simulink model "r2_c8n856m1k_wo_pfb"  (R2013a)
(part 2 of 31)

      | elseif strcmp(mode, 'fields of arbitrary size')
      |     current_names = textscan(strtrim(strrep(strrep(get_param(blk, 'names'), ']', ''), '[', '')), '%s');
      |     current_names = current_names{1};
      |     numios = length(current_names);
      |     if length(current_types) ~= numios,
      |         error('%d field names specified, but %d types?', numios, length(current_types));
      |     end
      | end
      | problem = 0;
      | for ctr = 1 : numios,
      |     t = current_types(ctr);
      |     if (t < 0) || (t > 2),
      |         problem = t;
      |         ctr = numios + 1;
      |     end
      | end
      | if problem ~= 0,
      |     error('Type cannot be %i, must be 0, 1 or 2.', problem);
      | end
      mask Callback bin_pts:
      | blk = gcb;
      | mode = get_param(blk, 'mode');
      | current_bins = eval(get_param(blk, 'bin_pts'));
      | if (strcmp(mode, 'one value') || strcmp(mode, 'fields of equal size')) && (length(current_bins) > 1),
      |     error('Only one binary pt may be specified for this mode.');
      | elseif strcmp(mode, 'fields of arbitrary size')
      |     current_names = textscan(strtrim(strrep(strrep(get_param(blk, 'names'), ']', ''), '[', '')), '%s');
      |     current_names = current_names{1};
      |     numios = length(current_names);
      |     if length(current_bins) ~= numios,
      |         error('%d field names specified, but %d binary pts?', numios, length(current_bins));
      |     end
      | end
  sync_timestamp_msw : Subsystem  Tag=xps:sw_reg  AncestorBlock=xps_library/software register  mask(swreg){mode=one value, io_dir=To Processor, io_delay=0, sample_period=1, names=reg, bitwidths=32, arith_types=0, bin_pts=0, sim_port=off, show_format=on}
      mask prompts: io_dir "I/O direction"; io_delay "I/O delay"; sample_period "Sample period"; names "Name:"; bitwidths "Bitwidth:"; arith_types "Type (ufix=0, fix=1, bool=2):"; bin_pts "Binary pt:"; sim_port "Provide sim input/output?"; show_format "Print format string?"
      mask init:
      | swreg_init(gcb)
      settings: AttributesFormatString=1output:uf32.0,
      mask TypeOptions mode: one value | fields of equal size | fields of arbitrary size
      mask Callback mode: swreg_cb(gcb);
      mask TypeOptions io_dir: To Processor | From Processor
      mask Callback io_dir:
      | mask_enables = get_param(gcb, 'MaskEnables');
      | mask_names = get_param(gcb, 'MaskNames');
      | if strcmp(get_param(gcb, 'io_dir'), 'To Processor'),
      |     mask_enables{ismember(mask_names, 'sample_period')} = 'off';
      | else
      |     mask_enables{ismember(mask_names, 'sample_period')} = 'on';
      | end
      | set_param(gcb, 'MaskEnables', mask_enables);
      mask Callback bitwidths:
      | blk = gcb;
      | mode = get_param(blk, 'mode');
      | current_widths = eval(get_param(blk, 'bitwidths'));
      | if (strcmp(mode, 'one value') || strcmp(mode, 'fields of equal size')) && (length(current_widths) > 1),
      |     error('Only one width may be specified for this mode.');
      | elseif strcmp(mode, 'fields of arbitrary size')
      |     current_names = textscan(strtrim(strrep(strrep(get_param(blk, 'names'), ']', ''), '[', '')), '%s');
      |     current_names = current_names{1};
      |     numios = length(current_names);
      |     if length(current_widths) ~= numios,
      |         error('%d field names specified, but %d widths?', numios, length(current_widths));
      |     end
      | end
      | total_width = 0;
      | for ctr = 1 : length(current_widths),
      |     total_width = total_width + current_widths(ctr);
      | end
      | if total_width > 32,
      |     error('Total width must be 32 or less, set to %d.', total_width);
      | end
      mask Callback arith_types:
      | blk = gcb;
      | mode = get_param(blk, 'mode');
      | current_types = eval(get_param(blk, 'arith_types'));
      | numios = length(current_types);
      | if (strcmp(mode, 'one value') || strcmp(mode, 'fields of equal size')) && (length(current_types) > 1),
      |     error('Only one type may be specified for this mode.');
      | elseif strcmp(mode, 'fields of arbitrary size')
      |     current_names = textscan(strtrim(strrep(strrep(get_param(blk, 'names'), ']', ''), '[', '')), '%s');
      |     current_names = current_names{1};
      |     numios = length(current_names);
      |     if length(current_types) ~= numios,
      |         error('%d field names specified, but %d types?', numios, length(current_types));
      |     end
      | end
      | problem = 0;
      | for ctr = 1 : numios,
      |     t = current_types(ctr);
      |     if (t < 0) || (t > 2),
      |         problem = t;
      |         ctr = numios + 1;
      |     end
      | end
      | if problem ~= 0,
      |     error('Type cannot be %i, must be 0, 1 or 2.', problem);
      | end
      mask Callback bin_pts:
      | blk = gcb;
      | mode = get_param(blk, 'mode');
      | current_bins = eval(get_param(blk, 'bin_pts'));
      | if (strcmp(mode, 'one value') || strcmp(mode, 'fields of equal size')) && (length(current_bins) > 1),
      |     error('Only one binary pt may be specified for this mode.');
      | elseif strcmp(mode, 'fields of arbitrary size')
      |     current_names = textscan(strtrim(strrep(strrep(get_param(blk, 'names'), ']', ''), '[', '')), '%s');
      |     current_names = current_names{1};
      |     numios = length(current_names);
      |     if length(current_bins) ~= numios,
      |         error('%d field names specified, but %d binary pts?', numios, length(current_bins));
      |     end
      | end
  timestep_ages : Subsystem  Tag=xps:sw_reg  AncestorBlock=xps_library/software register  mask(swreg){mode=fields of equal size, io_dir=To Processor, io_delay=0, sample_period=1, names=[future past], bitwidths=16, arith_types=0, bin_pts=0, sim_port=off, show_format=on}
      mask prompts: io_dir "I/O direction"; io_delay "I/O delay"; sample_period "Sample period"; names "Names [msb ... lsb]:"; bitwidths "Bitwidth:"; arith_types "Type (ufix=0, fix=1, bool=2):"; bin_pts "Binary pt:"; sim_port "Provide sim input/output?"; show_format "Print format string?"
      mask init:
      | swreg_init(gcb)
      settings: AttributesFormatString=2 outputs:uf16.0,uf16.0,
      mask TypeOptions mode: one value | fields of equal size | fields of arbitrary size
      mask Callback mode: swreg_cb(gcb);
      mask TypeOptions io_dir: To Processor | From Processor
      mask Callback io_dir:
      | mask_enables = get_param(gcb, 'MaskEnables');
      | mask_names = get_param(gcb, 'MaskNames');
      | if strcmp(get_param(gcb, 'io_dir'), 'To Processor'),
      |     mask_enables{ismember(mask_names, 'sample_period')} = 'off';
      | else
      |     mask_enables{ismember(mask_names, 'sample_period')} = 'on';
      | end
      | set_param(gcb, 'MaskEnables', mask_enables);
      mask Callback bitwidths:
      | blk = gcb;
      | mode = get_param(blk, 'mode');
      | current_widths = eval(get_param(blk, 'bitwidths'));
      | if (strcmp(mode, 'one value') || strcmp(mode, 'fields of equal size')) && (length(current_widths) > 1),
      |     error('Only one width may be specified for this mode.');
      | elseif strcmp(mode, 'fields of arbitrary size')
      |     current_names = textscan(strtrim(strrep(strrep(get_param(blk, 'names'), ']', ''), '[', '')), '%s');
      |     current_names = current_names{1};
      |     numios = length(current_names);
      |     if length(current_widths) ~= numios,
      |         error('%d field names specified, but %d widths?', numios, length(current_widths));
      |     end
      | end
      | total_width = 0;
      | for ctr = 1 : length(current_widths),
      |     total_width = total_width + current_widths(ctr);
      | end
      | if total_width > 32,
      |     error('Total width must be 32 or less, set to %d.', total_width);
      | end
      mask Callback arith_types:
      | blk = gcb;
      | mode = get_param(blk, 'mode');
      | current_types = eval(get_param(blk, 'arith_types'));
      | numios = length(current_types);
      | if (strcmp(mode, 'one value') || strcmp(mode, 'fields of equal size')) && (length(current_types) > 1),
      |     error('Only one type may be specified for this mode.');
      | elseif strcmp(mode, 'fields of arbitrary size')
      |     current_names = textscan(strtrim(strrep(strrep(get_param(blk, 'names'), ']', ''), '[', '')), '%s');
      |     current_names = current_names{1};
      |     numios = length(current_names);
      |     if length(current_types) ~= numios,
      |         error('%d field names specified, but %d types?', numios, length(current_types));
      |     end
      | end
      | problem = 0;
      | for ctr = 1 : numios,
      |     t = current_types(ctr);
      |     if (t < 0) || (t > 2),
      |         problem = t;
      |         ctr = numios + 1;
      |     end
      | end
      | if problem ~= 0,
      |     error('Type cannot be %i, must be 0, 1 or 2.', problem);
      | end
      mask Callback bin_pts:
      | blk = gcb;
      | mode = get_param(blk, 'mode');
      | current_bins = eval(get_param(blk, 'bin_pts'));
      | if (strcmp(mode, 'one value') || strcmp(mode, 'fields of equal size')) && (length(current_bins) > 1),
      |     error('Only one binary pt may be specified for this mode.');
      | elseif strcmp(mode, 'fields of arbitrary size')
      |     current_names = textscan(strtrim(strrep(strrep(get_param(blk, 'names'), ']', ''), '[', '')), '%s');
      |     current_names = current_names{1};
      |     numios = length(current_names);
      |     if length(current_bins) ~= numios,
      |         error('%d field names specified, but %d binary pts?', numios, length(current_bins));
      |     end
      | end
  tl_unpack_flags : Subsystem  mask(timed_latch){n_bits_time=48, n_bits_offset=(9+3), n_bits_counters=8}
      mask prompts: n_bits_time "Total time resolution (bits)"; n_bits_offset "Offset from lsb for comparison"; n_bits_counters "Bits in status counters"
      mask help:
      | Latches load_value when armed and current_time matches requested time.
      | current_time should be in ADC samples.
      mask init:
      | set_param([gcb,'/status'], 'bitwidths', mat2str([1, repmat(n_bits_counters, 1, 2)]));
      mask Help:
      | When armed, will latch new value when current time matches the time
      | specified. The input time should be in samples and mask settings allow
      | a portion of this to be compared to cater for quantization. Arm and latch
      | counts allow the current state, pending and missed latch events to be
      | determined.
  tmiss_ctr : Subsystem  Tag=xps:sw_reg  AncestorBlock=xps_library/software register  mask(swreg){mode=fields of equal size, io_dir=To Processor, io_delay=0, sample_period=1, names=[p0 p1], bitwidths=16, arith_types=0, bin_pts=0, sim_port=off, show_format=on}
      mask prompts: io_dir "I/O direction"; io_delay "I/O delay"; sample_period "Sample period"; names "Names [msb ... lsb]:"; bitwidths "Bitwidth:"; arith_types "Type (ufix=0, fix=1, bool=2):"; bin_pts "Binary pt:"; sim_port "Provide sim input/output?"; show_format "Print format string?"
      mask init:
      | swreg_init(gcb)
      settings: AttributesFormatString=2 outputs:uf16.0,uf16.0,
      mask TypeOptions mode: one value | fields of equal size | fields of arbitrary size
      mask Callback mode: swreg_cb(gcb);
      mask TypeOptions io_dir: To Processor | From Processor
      mask Callback io_dir:
      | mask_enables = get_param(gcb, 'MaskEnables');
      | mask_names = get_param(gcb, 'MaskNames');
      | if strcmp(get_param(gcb, 'io_dir'), 'To Processor'),
      |     mask_enables{ismember(mask_names, 'sample_period')} = 'off';
      | else
      |     mask_enables{ismember(mask_names, 'sample_period')} = 'on';
      | end
      | set_param(gcb, 'MaskEnables', mask_enables);
      mask Callback bitwidths:
      | blk = gcb;
      | mode = get_param(blk, 'mode');
      | current_widths = eval(get_param(blk, 'bitwidths'));
      | if (strcmp(mode, 'one value') || strcmp(mode, 'fields of equal size')) && (length(current_widths) > 1),
      |     error('Only one width may be specified for this mode.');
      | elseif strcmp(mode, 'fields of arbitrary size')
      |     current_names = textscan(strtrim(strrep(strrep(get_param(blk, 'names'), ']', ''), '[', '')), '%s');
      |     current_names = current_names{1};
      |     numios = length(current_names);
      |     if length(current_widths) ~= numios,
      |         error('%d field names specified, but %d widths?', numios, length(current_widths));
      |     end
      | end
      | total_width = 0;
      | for ctr = 1 : length(current_widths),
      |     total_width = total_width + current_widths(ctr);
      | end
      | if total_width > 32,
      |     error('Total width must be 32 or less, set to %d.', total_width);
      | end
      mask Callback arith_types:
      | blk = gcb;
      | mode = get_param(blk, 'mode');
      | current_types = eval(get_param(blk, 'arith_types'));
      | numios = length(current_types);
      | if (strcmp(mode, 'one value') || strcmp(mode, 'fields of equal size')) && (length(current_types) > 1),
      |     error('Only one type may be specified for this mode.');
      | elseif strcmp(mode, 'fields of arbitrary size')
      |     current_names = textscan(strtrim(strrep(strrep(get_param(blk, 'names'), ']', ''), '[', '')), '%s');
      |     current_names = current_names{1};
      |     numios = length(current_names);
      |     if length(current_types) ~= numios,
      |         error('%d field names specified, but %d types?', numios, length(current_types));
      |     end
      | end
      | problem = 0;
      | for ctr = 1 : numios,
      |     t = current_types(ctr);
      |     if (t < 0) || (t > 2),
      |         problem = t;
      |         ctr = numios + 1;
      |     end
      | end
      | if problem ~= 0,
      |     error('Type cannot be %i, must be 0, 1 or 2.', problem);
      | end
      mask Callback bin_pts:
      | blk = gcb;
      | mode = get_param(blk, 'mode');
      | current_bins = eval(get_param(blk, 'bin_pts'));
      | if (strcmp(mode, 'one value') || strcmp(mode, 'fields of equal size')) && (length(current_bins) > 1),
      |     error('Only one binary pt may be specified for this mode.');
      | elseif strcmp(mode, 'fields of arbitrary size')
      |     current_names = textscan(strtrim(strrep(strrep(get_param(blk, 'names'), ']', ''), '[', '')), '%s');
      |     current_names = current_names{1};
      |     numios = length(current_names);
      |     if length(current_bins) ~= numios,
      |         error('%d field names specified, but %d binary pts?', numios, length(current_bins));
      |     end
      | end
  tmiss_p0 : Subsystem  Tag=xps:sw_reg  AncestorBlock=xps_library/software register  mask(swreg){mode=one value, io_dir=To Processor, io_delay=0, sample_period=1, names=reg, bitwidths=32, arith_types=0, bin_pts=0, sim_port=off, show_format=on}
      mask prompts: io_dir "I/O direction"; io_delay "I/O delay"; sample_period "Sample period"; names "Name:"; bitwidths "Bitwidth:"; arith_types "Type (ufix=0, fix=1, bool=2):"; bin_pts "Binary pt:"; sim_port "Provide sim input/output?"; show_format "Print format string?"
      mask init:
      | swreg_init(gcb)
      settings: AttributesFormatString=1output:uf32.0,
      mask TypeOptions mode: one value | fields of equal size | fields of arbitrary size
      mask Callback mode: swreg_cb(gcb);
      mask TypeOptions io_dir: To Processor | From Processor
      mask Callback io_dir:
      | mask_enables = get_param(gcb, 'MaskEnables');
      | mask_names = get_param(gcb, 'MaskNames');
      | if strcmp(get_param(gcb, 'io_dir'), 'To Processor'),
      |     mask_enables{ismember(mask_names, 'sample_period')} = 'off';
      | else
      |     mask_enables{ismember(mask_names, 'sample_period')} = 'on';
      | end
      | set_param(gcb, 'MaskEnables', mask_enables);
      mask Callback bitwidths:
      | blk = gcb;
      | mode = get_param(blk, 'mode');
      | current_widths = eval(get_param(blk, 'bitwidths'));
      | if (strcmp(mode, 'one value') || strcmp(mode, 'fields of equal size')) && (length(current_widths) > 1),
      |     error('Only one width may be specified for this mode.');
      | elseif strcmp(mode, 'fields of arbitrary size')
      |     current_names = textscan(strtrim(strrep(strrep(get_param(blk, 'names'), ']', ''), '[', '')), '%s');
      |     current_names = current_names{1};
      |     numios = length(current_names);
      |     if length(current_widths) ~= numios,
      |         error('%d field names specified, but %d widths?', numios, length(current_widths));
      |     end
      | end
      | total_width = 0;
      | for ctr = 1 : length(current_widths),
      |     total_width = total_width + current_widths(ctr);
      | end
      | if total_width > 32,
      |     error('Total width must be 32 or less, set to %d.', total_width);
      | end
      mask Callback arith_types:
      | blk = gcb;
      | mode = get_param(blk, 'mode');
      | current_types = eval(get_param(blk, 'arith_types'));
      | numios = length(current_types);
      | if (strcmp(mode, 'one value') || strcmp(mode, 'fields of equal size')) && (length(current_types) > 1),
      |     error('Only one type may be specified for this mode.');
      | elseif strcmp(mode, 'fields of arbitrary size')
      |     current_names = textscan(strtrim(strrep(strrep(get_param(blk, 'names'), ']', ''), '[', '')), '%s');
      |     current_names = current_names{1};
      |     numios = length(current_names);
      |     if length(current_types) ~= numios,
      |         error('%d field names specified, but %d types?', numios, length(current_types));
      |     end
      | end
      | problem = 0;
      | for ctr = 1 : numios,
      |     t = current_types(ctr);
      |     if (t < 0) || (t > 2),
      |         problem = t;
      |         ctr = numios + 1;
      |     end
      | end
      | if problem ~= 0,
      |     error('Type cannot be %i, must be 0, 1 or 2.', problem);
      | end
      mask Callback bin_pts:
      | blk = gcb;
      | mode = get_param(blk, 'mode');
      | current_bins = eval(get_param(blk, 'bin_pts'));
      | if (strcmp(mode, 'one value') || strcmp(mode, 'fields of equal size')) && (length(current_bins) > 1),
      |     error('Only one binary pt may be specified for this mode.');
      | elseif strcmp(mode, 'fields of arbitrary size')
      |     current_names = textscan(strtrim(strrep(strrep(get_param(blk, 'names'), ']', ''), '[', '')), '%s');
      |     current_names = current_names{1};
      |     numios = length(current_names);
      |     if length(current_bins) ~= numios,
      |         error('%d field names specified, but %d binary pts?', numios, length(current_bins));
      |     end
      | end
  tmiss_p1 : Subsystem  Tag=xps:sw_reg  AncestorBlock=xps_library/software register  mask(swreg){mode=one value, io_dir=To Processor, io_delay=0, sample_period=1, names=reg, bitwidths=32, arith_types=0, bin_pts=0, sim_port=off, show_format=on}
      mask prompts: io_dir "I/O direction"; io_delay "I/O delay"; sample_period "Sample period"; names "Name:"; bitwidths "Bitwidth:"; arith_types "Type (ufix=0, fix=1, bool=2):"; bin_pts "Binary pt:"; sim_port "Provide sim input/output?"; show_format "Print format string?"
      mask init:
      | swreg_init(gcb)
      settings: AttributesFormatString=1output:uf32.0,
      mask TypeOptions mode: one value | fields of equal size | fields of arbitrary size
      mask Callback mode: swreg_cb(gcb);
      mask TypeOptions io_dir: To Processor | From Processor
      mask Callback io_dir:
      | mask_enables = get_param(gcb, 'MaskEnables');
      | mask_names = get_param(gcb, 'MaskNames');
      | if strcmp(get_param(gcb, 'io_dir'), 'To Processor'),
      |     mask_enables{ismember(mask_names, 'sample_period')} = 'off';
      | else
      |     mask_enables{ismember(mask_names, 'sample_period')} = 'on';
      | end
      | set_param(gcb, 'MaskEnables', mask_enables);
      mask Callback bitwidths:
      | blk = gcb;
      | mode = get_param(blk, 'mode');
      | current_widths = eval(get_param(blk, 'bitwidths'));
      | if (strcmp(mode, 'one value') || strcmp(mode, 'fields of equal size')) && (length(current_widths) > 1),
      |     error('Only one width may be specified for this mode.');
      | elseif strcmp(mode, 'fields of arbitrary size')
      |     current_names = textscan(strtrim(strrep(strrep(get_param(blk, 'names'), ']', ''), '[', '')), '%s');
      |     current_names = current_names{1};
      |     numios = length(current_names);
      |     if length(current_widths) ~= numios,
      |         error('%d field names specified, but %d widths?', numios, length(current_widths));
      |     end
      | end
      | total_width = 0;
      | for ctr = 1 : length(current_widths),
      |     total_width = total_width + current_widths(ctr);
      | end
      | if total_width > 32,
      |     error('Total width must be 32 or less, set to %d.', total_width);
      | end
      mask Callback arith_types:
      | blk = gcb;
      | mode = get_param(blk, 'mode');
      | current_types = eval(get_param(blk, 'arith_types'));
      | numios = length(current_types);
      | if (strcmp(mode, 'one value') || strcmp(mode, 'fields of equal size')) && (length(current_types) > 1),
      |     error('Only one type may be specified for this mode.');
      | elseif strcmp(mode, 'fields of arbitrary size')
      |     current_names = textscan(strtrim(strrep(strrep(get_param(blk, 'names'), ']', ''), '[', '')), '%s');
      |     current_names = current_names{1};
      |     numios = length(current_names);
      |     if length(current_types) ~= numios,
      |         error('%d field names specified, but %d types?', numios, length(current_types));
      |     end
      | end
      | problem = 0;
      | for ctr = 1 : numios,
      |     t = current_types(ctr);
      |     if (t < 0) || (t > 2),
      |         problem = t;
      |         ctr = numios + 1;
      |     end
      | end
      | if problem ~= 0,
      |     error('Type cannot be %i, must be 0, 1 or 2.', problem);
      | end
      mask Callback bin_pts:
      | blk = gcb;
      | mode = get_param(blk, 'mode');
      | current_bins = eval(get_param(blk, 'bin_pts'));
      | if (strcmp(mode, 'one value') || strcmp(mode, 'fields of equal size')) && (length(current_bins) > 1),
      |     error('Only one binary pt may be specified for this mode.');
      | elseif strcmp(mode, 'fields of arbitrary size')
      |     current_names = textscan(strtrim(strrep(strrep(get_param(blk, 'names'), ']', ''), '[', '')), '%s');
      |     current_names = current_names{1};
      |     numios = length(current_names);
      |     if length(current_bins) ~= numios,
      |         error('%d field names specified, but %d binary pts?', numios, length(current_bins));
      |     end
      | end
  trig0 : Subsystem  mask{mult_latency=3}
      mask prompts: mult_latency "Multiplier latency"
  trig1 : Subsystem  mask{mult_latency=3}
      mask prompts: mult_latency "Multiplier latency"
  trigger_level : Subsystem  Tag=xps:sw_reg  AncestorBlock=xps_library/software register  mask(swreg){mode=one value, io_dir=From Processor, io_delay=0, sample_period=1, names=trigger_level, bitwidths=32, arith_types=0, bin_pts=0, show_format=off}
      mask prompts: io_dir "I/O direction"; io_delay "I/O delay"; sample_period "Sample period"; names "Name:"; bitwidths "Bitwidth:"; arith_types "Type (ufix=0, fix=1, bool=2):"; bin_pts "Binary pt:"; show_format "Print format string?"
      mask init:
      | swreg_init(gcb)
      settings: AttributesFormatString=1input
      mask TypeOptions mode: one value | fields of equal size | fields of arbitrary size
      mask Callback mode: swreg_cb(gcb);
      mask TypeOptions io_dir: To Processor | From Processor
      mask Callback io_dir:
      | mask_enables = get_param(gcb, 'MaskEnables');
      | mask_names = get_param(gcb, 'MaskNames');
      | if strcmp(get_param(gcb, 'io_dir'), 'To Processor'),
      |     mask_enables{ismember(mask_names, 'sample_period')} = 'off';
      | else
      |     mask_enables{ismember(mask_names, 'sample_period')} = 'on';
      | end
      | set_param(gcb, 'MaskEnables', mask_enables);
      mask Callback bitwidths:
      | blk = gcb;
      | mode = get_param(blk, 'mode');
      | current_widths = eval(get_param(blk, 'bitwidths'));
      | if (strcmp(mode, 'one value') || strcmp(mode, 'fields of equal size')) && (length(current_widths) > 1),
      |     error('Only one width may be specified for this mode.');
      | elseif strcmp(mode, 'fields of arbitrary size')
      |     current_names = textscan(strtrim(strrep(strrep(get_param(blk, 'names'), ']', ''), '[', '')), '%s');
      |     current_names = current_names{1};
      |     numios = length(current_names);
      |     if length(current_widths) ~= numios,
      |         error('%d field names specified, but %d widths?', numios, length(current_widths));
      |     end
      | end
      | total_width = 0;
      | for ctr = 1 : length(current_widths),
      |     total_width = total_width + current_widths(ctr);
      | end
      | if total_width > 32,
      |     error('Total width must be 32 or less, set to %d.', total_width);
      | end
      mask Callback arith_types:
      | blk = gcb;
      | mode = get_param(blk, 'mode');
      | current_types = eval(get_param(blk, 'arith_types'));
      | numios = length(current_types);
      | if (strcmp(mode, 'one value') || strcmp(mode, 'fields of equal size')) && (length(current_types) > 1),
      |     error('Only one type may be specified for this mode.');
      | elseif strcmp(mode, 'fields of arbitrary size')
      |     current_names = textscan(strtrim(strrep(strrep(get_param(blk, 'names'), ']', ''), '[', '')), '%s');
      |     current_names = current_names{1};
      |     numios = length(current_names);
      |     if length(current_types) ~= numios,
      |         error('%d field names specified, but %d types?', numios, length(current_types));
      |     end
      | end
      | problem = 0;
      | for ctr = 1 : numios,
      |     t = current_types(ctr);
      |     if (t < 0) || (t > 2),
      |         problem = t;
      |         ctr = numios + 1;
      |     end
      | end
      | if problem ~= 0,
      |     error('Type cannot be %i, must be 0, 1 or 2.', problem);
      | end
      mask Callback bin_pts:
      | blk = gcb;
      | mode = get_param(blk, 'mode');
      | current_bins = eval(get_param(blk, 'bin_pts'));
      | if (strcmp(mode, 'one value') || strcmp(mode, 'fields of equal size')) && (length(current_bins) > 1),
      |     error('Only one binary pt may be specified for this mode.');
      | elseif strcmp(mode, 'fields of arbitrary size')
      |     current_names = textscan(strtrim(strrep(strrep(get_param(blk, 'names'), ']', ''), '[', '')), '%s');
      |     current_names = current_names{1};
      |     numios = length(current_names);
      |     if length(current_bins) ~= numios,
      |         error('%d field names specified, but %d binary pts?', numios, length(current_bins));
      |     end
      | end
  tx_metadata : Subsystem  Tag=xps:sw_reg  AncestorBlock=xps_library/software register  mask(swreg){mode=fields of arbitrary size, io_dir=From Processor, io_delay=0, sample_period=1, names=[porttx board_id], bitwidths=16, arith_types=0, bin_pts=0, sim_port=on, show_format=off}
      mask prompts: io_dir "I/O direction"; io_delay "I/O delay"; sample_period "Sample period"; names "Names [msb ... lsb]:"; bitwidths "Bitwidths [msb ... lsb]:"; arith_types "Types (ufix=0, fix=1, bool=2) [msb ... lsb]:"; bin_pts "Binary pts [msb ... lsb]:"; sim_port "Provide sim input/output?"; show_format "Print format string?"
      mask init:
      | swreg_init(gcb)
      settings: AttributesFormatString=2 inputs
      mask TypeOptions mode: one value | fields of equal size | fields of arbitrary size
      mask Callback mode: swreg_cb(gcb);
      mask TypeOptions io_dir: To Processor | From Processor
      mask Callback io_dir:
      | mask_enables = get_param(gcb, 'MaskEnables');
      | mask_names = get_param(gcb, 'MaskNames');
      | if strcmp(get_param(gcb, 'io_dir'), 'To Processor'),
      |     mask_enables{ismember(mask_names, 'sample_period')} = 'off';
      | else
      |     mask_enables{ismember(mask_names, 'sample_period')} = 'on';
      | end
      | set_param(gcb, 'MaskEnables', mask_enables);
      mask Callback bitwidths:
      | swreg_maskcheck(gcb);
      | % blk = gcb;
      | % mode = get_param(blk, 'mode');
      | % current_widths = eval(get_param(blk, 'bitwidths'));
      | % if (strcmp(mode, 'one value') || strcmp(mode, 'fields of equal size')) && (length(current_widths) > 1),
      | %     error('Only one width may be specified for this mode.');
      | % elseif strcmp(mode, 'fields of arbitrary size')
      | %     current_names = textscan(strtrim(strrep(strrep(get_param(blk, 'names'), ']', ''), '[', '')), '%s');
      | %     current_names = current_names{1};
      | %     numios = length(current_names);
      | %     if length(current_widths) ~= numios,
      | %         error('%d field names specified, but %d widths?', numios, length(current_widths));
      | %     end
      | % end
      | % total_width = 0;
      | % for ctr = 1 : length(current_widths),
      | %     total_width = total_width + current_widths(ctr);
      | % end
      | % if total_width > 32,
      | %     error('Total width must be 32 or less, set to %d.', total_width);
      | % end
      mask Callback arith_types:
      | [numios, ~, ~, ~, current_types] = swreg_maskcheck(gcb);
      | % blk = gcb;
      | % mode = get_param(blk, 'mode');
      | % current_types = eval(get_param(blk, 'arith_types'));
      | % numios = length(current_types);
      | % if (strcmp(mode, 'one value') || strcmp(mode, 'fields of equal size')) && (length(current_types) > 1),
      | %     error('Only one type may be specified for this mode.');
      | % elseif strcmp(mode, 'fields of arbitrary size')
      | %     current_names = textscan(strtrim(strrep(strrep(get_param(blk, 'names'), ']', ''), '[', '')), '%s');
      | %     current_names = current_names{1};
      | %     numios = length(current_names);
      | %     if length(current_types) ~= numios,
      | %         error('%d field names specified, but %d types?', numios, length(current_types));
      | %     end
      | % end
      | problem = 0;
      | for ctr = 1 : numios,
      |     t = current_types(ctr);
      |     if (t < 0) || (t > 2),
      |         problem = t;
      |         ctr = numios + 1;
      |     end
      | end
      | if problem ~= 0,
      |     error('Type cannot be %i, must be 0, 1 or 2.', problem);
      | end
      mask Callback bin_pts:
      | swreg_maskcheck(gcb);
      | % blk = gcb;
      | % mode = get_param(blk, 'mode');
      | % current_bins = eval(get_param(blk, 'bin_pts'));
      | % if (strcmp(mode, 'one value') || strcmp(mode, 'fields of equal size')) && (length(current_bins) > 1),
      | %     error('Only one binary pt may be specified for this mode.');
      | % elseif strcmp(mode, 'fields of arbitrary size')
      | %     current_names = textscan(strtrim(strrep(strrep(get_param(blk, 'names'), ']', ''), '[', '')), '%s');
      | %     current_names = current_names{1};
      | %     numios = length(current_names);
      | %     if length(current_bins) ~= numios,
      | %         error('%d field names specified, but %d binary pts?', numios, length(current_bins));
      | %     end
      | % end
  unpack_and_reorder : Subsystem  mask{n_bits_packet_size=9, n_bits_timestep=9+3, n_bits_fifo_depth=3, n_bits_buffer_depth=3, bram_latency=1}
      mask prompts: n_bits_packet_size "Packet size (2^? 80-bit words after unpacking)"; n_bits_timestep "Packet timestep (2^?)"; n_bits_fifo_depth "FIFO depth (2^? packets)"; n_bits_buffer_depth "Reorder buffer size (2^? packets)"; bram_latency "BRAM latency"
  unpack_flags : Subsystem  Tag=xps:sw_reg  AncestorBlock=xps_library/software register  mask(swreg){mode=fields of arbitrary size, io_dir=From Processor, io_delay=1, sample_period=1, names=[timestep_error missing0 missing1 mcnt_relock discarded pktof fifo_of spead_error adc_or0 adc_or1 ndiode0 ndiode1], bitwidths=[1 1 1 1 1 1 1 1 1 1 1 1], arith_types=[0 0 0 0 0 0 0 0 0 0 0 0], bin_pts=[0 0 0 0 0 0 0 0 0 0 0 0], sim_port=off, show_format=off}
      mask prompts: io_dir "I/O direction"; io_delay "I/O delay"; sample_period "Sample period"; names "Names [msb ... lsb]:"; bitwidths "Bitwidths [msb ... lsb]:"; arith_types "Types (ufix=0, fix=1, bool=2) [msb ... lsb]:"; bin_pts "Binary pts [msb ... lsb]:"; sim_port "Provide sim input/output?"; show_format "Print format string?"
      mask init:
      | swreg_init(gcb)
      settings: AttributesFormatString=12 inputs
      mask TypeOptions mode: one value | fields of equal size | fields of arbitrary size
      mask Callback mode: swreg_cb(gcb);
      mask TypeOptions io_dir: To Processor | From Processor
      mask Callback io_dir:
      | mask_enables = get_param(gcb, 'MaskEnables');
      | mask_names = get_param(gcb, 'MaskNames');
      | if strcmp(get_param(gcb, 'io_dir'), 'To Processor'),
      |     mask_enables{ismember(mask_names, 'sample_period')} = 'off';
      | else
      |     mask_enables{ismember(mask_names, 'sample_period')} = 'on';
      | end
      | set_param(gcb, 'MaskEnables', mask_enables);
      mask Callback bitwidths:
      | swreg_maskcheck(gcb);
      | % blk = gcb;
      | % mode = get_param(blk, 'mode');
      | % current_widths = eval(get_param(blk, 'bitwidths'));
      | % if (strcmp(mode, 'one value') || strcmp(mode, 'fields of equal size')) && (length(current_widths) > 1),
      | %     error('Only one width may be specified for this mode.');
      | % elseif strcmp(mode, 'fields of arbitrary size')
      | %     current_names = textscan(strtrim(strrep(strrep(get_param(blk, 'names'), ']', ''), '[', '')), '%s');
      | %     current_names = current_names{1};
      | %     numios = length(current_names);
      | %     if length(current_widths) ~= numios,
      | %         error('%d field names specified, but %d widths?', numios, length(current_widths));
      | %     end
      | % end
      | % total_width = 0;
      | % for ctr = 1 : length(current_widths),
      | %     total_width = total_width + current_widths(ctr);
      | % end
      | % if total_width > 32,
      | %     error('Total width must be 32 or less, set to %d.', total_width);
      | % end
      mask Callback arith_types:
      | [numios, ~, ~, ~, current_types] = swreg_maskcheck(gcb);
      | % blk = gcb;
      | % mode = get_param(blk, 'mode');
      | % current_types = eval(get_param(blk, 'arith_types'));
      | % numios = length(current_types);
      | % if (strcmp(mode, 'one value') || strcmp(mode, 'fields of equal size')) && (length(current_types) > 1),
      | %     error('Only one type may be specified for this mode.');
      | % elseif strcmp(mode, 'fields of arbitrary size')
      | %     current_names = textscan(strtrim(strrep(strrep(get_param(blk, 'names'), ']', ''), '[', '')), '%s');
      | %     current_names = current_names{1};
      | %     numios = length(current_names);
      | %     if length(current_types) ~= numios,
      | %         error('%d field names specified, but %d types?', numios, length(current_types));
      | %     end
      | % end
      | problem = 0;
      | for ctr = 1 : numios,
      |     t = current_types(ctr);
      |     if (t < 0) || (t > 2),
      |         problem = t;
      |         ctr = numios + 1;
      |     end
      | end
      | if problem ~= 0,
      |     error('Type cannot be %i, must be 0, 1 or 2.', problem);
      | end
      mask Callback bin_pts:
      | swreg_maskcheck(gcb);
      | % blk = gcb;
      | % mode = get_param(blk, 'mode');
      | % current_bins = eval(get_param(blk, 'bin_pts'));
      | % if (strcmp(mode, 'one value') || strcmp(mode, 'fields of equal size')) && (length(current_bins) > 1),
      | %     error('Only one binary pt may be specified for this mode.');
      | % elseif strcmp(mode, 'fields of arbitrary size')
      | %     current_names = textscan(strtrim(strrep(strrep(get_param(blk, 'names'), ']', ''), '[', '')), '%s');
      | %     current_names = current_names{1};
      | %     numios = length(current_names);
      | %     if length(current_bins) ~= numios,
      | %         error('%d field names specified, but %d binary pts?', numios, length(current_bins));
      | %     end
      | % end
  up_debug : Subsystem  Tag=xps:sw_reg  AncestorBlock=xps_library/software register  mask(swreg){mode=one value, io_dir=From Processor, io_delay=0, sample_period=1, names=gbe_timestep, bitwidths=3, arith_types=0, bin_pts=0, sim_port=off, show_format=on}
      mask prompts: io_dir "I/O direction"; io_delay "I/O delay"; sample_period "Sample period"; names "Name:"; bitwidths "Bitwidth:"; arith_types "Type (ufix=0, fix=1, bool=2):"; bin_pts "Binary pt:"; sim_port "Provide sim input/output?"; show_format "Print format string?"
      mask init:
      | swreg_init(gcb)
      settings: AttributesFormatString=1input:uf3.0,
      mask TypeOptions mode: one value | fields of equal size | fields of arbitrary size
      mask Callback mode: swreg_cb(gcb);
      mask TypeOptions io_dir: To Processor | From Processor
      mask Callback io_dir:
      | mask_enables = get_param(gcb, 'MaskEnables');
      | mask_names = get_param(gcb, 'MaskNames');
      | if strcmp(get_param(gcb, 'io_dir'), 'To Processor'),
      |     mask_enables{ismember(mask_names, 'sample_period')} = 'off';
      | else
      |     mask_enables{ismember(mask_names, 'sample_period')} = 'on';
      | end
      | set_param(gcb, 'MaskEnables', mask_enables);
      mask Callback bitwidths:
      | blk = gcb;
      | mode = get_param(blk, 'mode');
      | current_widths = eval(get_param(blk, 'bitwidths'));
      | if (strcmp(mode, 'one value') || strcmp(mode, 'fields of equal size')) && (length(current_widths) > 1),
      |     error('Only one width may be specified for this mode.');
      | elseif strcmp(mode, 'fields of arbitrary size')
      |     current_names = textscan(strtrim(strrep(strrep(get_param(blk, 'names'), ']', ''), '[', '')), '%s');
      |     current_names = current_names{1};
      |     numios = length(current_names);
      |     if length(current_widths) ~= numios,
      |         error('%d field names specified, but %d widths?', numios, length(current_widths));
      |     end
      | end
      | total_width = 0;
      | for ctr = 1 : length(current_widths),
      |     total_width = total_width + current_widths(ctr);
      | end
      | if total_width > 32,
      |     error('Total width must be 32 or less, set to %d.', total_width);
      | end
      mask Callback arith_types:
      | blk = gcb;
      | mode = get_param(blk, 'mode');
      | current_types = eval(get_param(blk, 'arith_types'));
      | numios = length(current_types);
      | if (strcmp(mode, 'one value') || strcmp(mode, 'fields of equal size')) && (length(current_types) > 1),
      |     error('Only one type may be specified for this mode.');
      | elseif strcmp(mode, 'fields of arbitrary size')
      |     current_names = textscan(strtrim(strrep(strrep(get_param(blk, 'names'), ']', ''), '[', '')), '%s');
      |     current_names = current_names{1};
      |     numios = length(current_names);
      |     if length(current_types) ~= numios,
      |         error('%d field names specified, but %d types?', numios, length(current_types));
      |     end
      | end
      | problem = 0;
      | for ctr = 1 : numios,
      |     t = current_types(ctr);
      |     if (t < 0) || (t > 2),
      |         problem = t;
      |         ctr = numios + 1;
      |     end
      | end
      | if problem ~= 0,
      |     error('Type cannot be %i, must be 0, 1 or 2.', problem);
      | end
      mask Callback bin_pts:
      | blk = gcb;
      | mode = get_param(blk, 'mode');
      | current_bins = eval(get_param(blk, 'bin_pts'));
      | if (strcmp(mode, 'one value') || strcmp(mode, 'fields of equal size')) && (length(current_bins) > 1),
      |     error('Only one binary pt may be specified for this mode.');
      | elseif strcmp(mode, 'fields of arbitrary size')
      |     current_names = textscan(strtrim(strrep(strrep(get_param(blk, 'names'), ']', ''), '[', '')), '%s');
      |     current_names = current_names{1};
      |     numios = length(current_names);
      |     if length(current_bins) ~= numios,
      |         error('%d field names specified, but %d binary pts?', numios, length(current_bins));
      |     end
      | end
  xps : xps_library/XSG core config  Tag=xps:xsg  hw_sys=ROACH2:sx475t  clk_src=sys_clk  ROACH_clk_src=adc0_clk  ROACH2_clk_src=sys_clk  MKDIG_clk_src=sys_clk  clk_rate=224  sample_period=1  synthesis_tool=XST
  tag scope: cnt_rst=global, gbe_timestep=global, tvg_pfb_flags_en=global, tvg_unpack_flags_en=global, up_cnt_rst=global, wintime_snap_wesel=global
  wires:
  gbe0/1(led_up) -> [up_gbe0]
  gbe0/2(led_rx) -> [rx_gbe0]
  gbe0/3(led_tx) -> [tx_gbe0]
  gbe0/5(tx_overflow) -> [tx_over_gbe0]
  gbe0/12(rx_overrun) -> [rxover_gbe0]
  gbe0/11(rx_bad_frame) -> [rxbad_gbe0]
  gbe0/6(rx_data) -> [rxdata_gbe0]
  gbe0/7(rx_valid) -> [rxvld_gbe0]
  gbe0/8(rx_source_ip) -> [rxip_gbe0]
  gbe0/9(rx_source_port) -> [rxport_gbe0]
  gbe0/10(rx_end_of_frame) -> [rxeof_gbe0]
  [gbe_rst] -> pipeline102/1(d)
  gbe1/1(led_up) -> [up_gbe1]
  gbe1/2(led_rx) -> [rx_gbe1]
  gbe1/3(led_tx) -> [tx_gbe1]
  gbe1/4(tx_afull) -> [tx_full_gbe1]
  gbe1/5(tx_overflow) -> [tx_over_gbe1]
  gbe1/12(rx_overrun) -> [rxover_gbe1]
  gbe1/11(rx_bad_frame) -> [rxbad_gbe1]
  gbe1/6(rx_data) -> [rxdata_gbe1]
  gbe1/7(rx_valid) -> [rxvld_gbe1]
  gbe1/8(rx_source_ip) -> [rxip_gbe1]
  gbe1/9(rx_source_port) -> [rxport_gbe1]
  gbe1/10(rx_end_of_frame) -> [rxeof_gbe1]
  gbe2/1(led_up) -> [up_gbe2]
  gbe2/2(led_rx) -> [rx_gbe2]
  gbe2/3(led_tx) -> [tx_gbe2]
  gbe2/4(tx_afull) -> [tx_full_gbe2]
  gbe2/5(tx_overflow) -> [tx_over_gbe2]
  gbe2/12(rx_overrun) -> [rxover_gbe2]
  gbe2/11(rx_bad_frame) -> [rxbad_gbe2]
  gbe2/6(rx_data) -> [rxdata_gbe2]
  gbe2/7(rx_valid) -> [rxvld_gbe2]
  gbe2/8(rx_source_ip) -> [rxip_gbe2]
  gbe2/9(rx_source_port) -> [rxport_gbe2]
  gbe2/10(rx_end_of_frame) -> [rxeof_gbe2]
  gbe3/1(led_up) -> [up_gbe3]
  gbe3/2(led_rx) -> [rx_gbe3]
  gbe3/3(led_tx) -> [tx_gbe3]
  gbe3/4(tx_afull) -> [tx_full_gbe3]
  gbe3/5(tx_overflow) -> [tx_over_gbe3]
  gbe3/12(rx_overrun) -> [rxover_gbe3]
  gbe3/11(rx_bad_frame) -> [rxbad_gbe3]
  gbe3/6(rx_data) -> [rxdata_gbe3]
  gbe3/7(rx_valid) -> [rxvld_gbe3]
  gbe3/8(rx_source_ip) -> [rxip_gbe3]
  gbe3/9(rx_source_port) -> [rxport_gbe3]
  gbe3/10(rx_end_of_frame) -> [rxeof_gbe3]
  gbe0/4(tx_afull) -> [tx_full_gbe0]
  edge_detect3/1(out) -> pipeline4/1(d)
  edge_detect4/1(out) -> pipeline3/1(d)
  edge_detect5/1(out) -> pipeline2/1(d)
  [sys_rst] -> edge_detect9/1(in)
  [rxdata_gbe0] -> concat0/1
  [rxdata_gbe1] -> concat0/2
  [rxdata_gbe2] -> concat0/3
  [rxdata_gbe3] -> concat0/4
  [rxeof_gbe0] -> concat1/1
  [rxeof_gbe1] -> concat1/2
  [rxeof_gbe2] -> concat1/3
  [rxeof_gbe3] -> concat1/4
  [rxvld_gbe0] -> concat3/1
  [rxvld_gbe1] -> concat3/2
  [rxvld_gbe2] -> concat3/3
  [rxvld_gbe3] -> concat3/4
  bus_expand2/4(lsb_out1) -> [unpack_adc_or1]
  control/2(in_arm) -> edge_detect5/1(in)
  control/13(in_cnt_rst) -> edge_detect1/1(in)
  concat0/1 -> pipeline31/1(d)
  concat1/1 -> pipeline62/1(d)
  concat3/1 -> pipeline63/1(d)
  constant/1 -> unpack_and_reorder/5(transmit)
  unpack_and_reorder/4(timestamp) -> [unpack_timestamp]
  unpack_and_reorder/5(recvd) -> bus_expand17/1(bus_in)
  unpack_and_reorder/1(sync) -> [unpack_sync]
  edge_detect1/1(out) -> pipeline14/1(d)
  control/4(in_gbe_rst) -> pipeline5/1(d)
  control/1(in_sys_rst) -> pipeline/1(d)
  Constant4/1 -> gbe1/8(rx_overrun_ack), gbe1/7(rx_ack)
  [gbe_rst] -> pipeline104/1(d)
  Constant23/1 -> gbe2/8(rx_overrun_ack), gbe2/7(rx_ack)
  [gbe_rst] -> pipeline103/1(d)
  Constant33/1 -> gbe3/8(rx_overrun_ack), gbe3/7(rx_ack)
  [gbe_rst] -> pipeline101/1(d)
  Constant20/1 -> gbe0/8(rx_overrun_ack), gbe0/7(rx_ack)
  [gbe_cnt_rst] -> pipeline93/1(d)
  [gbe_cnt_rst] -> pipeline100/1(d)
  [gbe_cnt_rst] -> pipeline98/1(d)
  [gbe_cnt_rst] -> pipeline99/1(d)
  Constant10/1 -> iptx_base/1(sim_1)
  Constant3/1 -> tx_metadata/1(sim_1)
  Constant5/1 -> tx_metadata/2(sim_2)
  pipeline/1(q) -> [sys_rst]
  pipeline2/1(q) -> [arm]
  pipeline3/1(q) -> [clr_status]
  pipeline4/1(q) -> [clr_adc_bad]
  pipeline5/1(q) -> [gbe_rst]
  pipeline6/1(q) -> [gbe_txen]
  pipeline8/1(q) -> [adc_protect_disable]
  pipeline9/1(q) -> [tvg_en]
  pipeline10/1(q) -> [ct_tvg]
  pipeline11/1(q) -> [packetiser_tvg]
  pipeline12/1(q) -> [fd_fs_tvg]
  pipeline13/1(q) -> [tvg_adc_en]
  pipeline14/1(q) -> [cnt_rst]
  control/12(in_tvg_adc) -> pipeline13/1(d)
  pipeline31/1(q) -> unpack_and_reorder/2(din)
  edge_detect2/1(out) -> pipeline7/1(d)
  pipeline7/1(q) -> [gbe_cnt_rst]
  control/14(in_gbe_cnt_rst) -> edge_detect2/1(in)
  edge_detect7/1(out) -> pipeline15/1(d)
  pipeline15/1(q) -> [up_cnt_rst]
  Constant/1 -> Delay10/1
  Constant7/1 -> Delay11/1
  Constant9/1 -> Delay12/1
  unpack_and_reorder/2(dout) -> [unpack_d80]
  unpack_and_reorder/3(dvalid) -> [unpack_en]
  unpack_and_reorder/10(discarding) -> [unpack_discarding]
  unpack_and_reorder/11(timestep_error) -> [timestep_error]
  Constant25/1 -> trigger_level/1(sim_1)
  [d80_adc1] -> trig1/2(adc_data)
  trig1/3(trig) -> [trans_stop_1]
  trig1/2(data) -> [trans_d80_1]
  trig0/2(data) -> [trans_d80_0]
  trig0/3(trig) -> [trans_stop_0]
  [d80_adc0] -> trig0/2(adc_data)
  trig1/1(synco) -> [trans_valid80]
  [sync80] -> Concat6/1
  [time80] -> Slice14/1
  Concat6/1 -> trig0/1(synci)
  trig0/1(synco) -> bus_expand/1(bus_in)
  bus_expand/1(msb_out2) -> [trans_trig]
  Slice14/1 -> Concat6/2
  bus_expand/2(lsb_out1) -> [trans_time]
  [valid80] -> trig1/1(synci)
  trigger_level/1(in_trigger_level) -> pipeline17/1(d)
  en_gen/1(dout) -> sync_gen/1(din)
  pipeline17/1(q) -> trig1/3(trig_pnt), trig0/3(trig_pnt)
  en_gen/3(time_out) -> sync_gen/3(time_in)
  en_gen/2(dvalid) -> sync_gen/2(en)
  en_gen/4(misco) -> sync_gen/4(misci), Slice20/1
  Slice20/1 -> sync_gen/5(relock)
  sync_gen/2(dout) -> bus_expand6/1(bus_in)
  sync_gen/3(dvalid) -> impulse_gen0/6(en), impulse_gen1/6(en)
  Slice/1 -> pipeline16/1(d)
  pipeline16/1(q) -> local_time_lsw/1(out_timestamp_lsw)
  Slice16/1 -> Convert1/1
  pipeline47/1(q) -> local_time_msw/1(out_timestamp_msw)
  Convert1/1 -> pipeline47/1(d)
  Concat2/1 -> Slice16/1, [time80_48], Slice/1
  [time80] -> Concat2/1
  Constant53/1 -> Concat2/2
  control/15(in_unpack_cnt_rst) -> edge_detect7/1(in)
  pipeline18/1(q) -> [snappfb_arm]
  control/17(in_snappfb_arm) -> pipeline18/1(d)
  control/5(in_gbe_txen) -> pipeline6/1(d)
  control/6(in_adc_bad_clr) -> edge_detect3/1(in)
  control/7(in_adc_protect_disable) -> pipeline8/1(d)
  control/8(in_tvg_en) -> pipeline9/1(d)
  control/9(in_tvg_ct) -> pipeline10/1(d)
  control/10(in_tvg_packetiser) -> pipeline11/1(d)
  control/11(in_tvg_fdfs) -> pipeline12/1(d)
  pipeline19/1(q) -> [tvg_d80_en]
  control/20(in_tvg_d80) -> pipeline19/1(d)
  control/3(in_status_clr) -> edge_detect4/1(in)
  Register11/1 -> Slice7/1, Slice9/1
  [time80] -> pipeline54/1(d)
  Slice7/1 -> pipeline112/1(d)
  [sync80] -> pipeline52/1(d)
  [valid80] -> pipeline53/1(d)
  Register12/1 -> Logical1/1  "armed"
  Logical1/1 -> Register12/2, Register11/2
  pipeline52/1(q) -> Register12/3, Register12/1
  pipeline53/1(q) -> Logical1/2
  pipeline54/1(q) -> Register11/1
  [valid80] -> pipeline55/1(d)
  pipeline55/1(q) -> Delay42/1, edge_detect13/1(in)
  counter8/1 -> Register13/1
  edge_detect13/1(out) -> counter8/1, Register13/2
  Delay42/1 -> counter8/2
  Slice9/1 -> pipeline113/1(d)
  Register13/1 -> pipeline114/1(d)
  pipeline56/1(q) -> edge_detect14/1(in)
  edge_detect14/1(out) -> counter9/2
  [timestep_error] -> pipeline56/1(d)
  [cnt_rst] -> pipeline57/1(d)
  pipeline57/1(q) -> counter9/1
  pipeline58/1(q) -> edge_detect15/1(in)
  edge_detect15/1(out) -> counter10/2
  [sync80] -> pipeline58/1(d)
  [cnt_rst] -> pipeline51/1(d)
  pipeline51/1(q) -> counter10/1
  pipeline59/1(q) -> edge_detect16/1(in)
  edge_detect16/1(out) -> counter11/2
  [valid80] -> pipeline59/1(d)
  [cnt_rst] -> pipeline60/1(d)
  pipeline60/1(q) -> counter11/1
  counter9/1 -> pipeline115/1(d)
  counter10/1 -> pipeline116/1(d)
  counter11/1 -> pipeline117/1(d)
  pipeline48/1(q) -> [wintime_snap_wesel]
  control/21(in_wintime_snap_wesel) -> pipeline48/1(d)
  edge_detect9/1(out) -> pipeline64/1(d)
  [up_p0_missed_time_ctr] -> Delay76/1(d)
  [up_p1_missed_time_ctr] -> Delay77/1(d)
  [up_p0_missed_time] -> Delay81/1(d)
  [up_p1_missed_time] -> Delay83/1(d)
  Delay81/1(q) -> Slice10/1
  Delay83/1(q) -> Slice11/1
  Delay76/1(q) -> tmiss_ctr/1(out_p0)
  Delay77/1(q) -> tmiss_ctr/2(out_p1)
  Inverter2/1 -> Logical5/1
  [unpack_en] -> Logical6/2, Logical5/2
  Logical5/1 -> counter20/2
  [cnt_rst] -> Delay79/1(d)
  counter20/1 -> Delay7/1(d)
  counter21/1 -> Delay13/1(d)
  [unpack_mcnt_relock] -> counter21/2
  Slice10/1 -> tmiss_p0/1(out_reg)
  Slice11/1 -> tmiss_p1/1(out_reg)
  counter22/1 -> Delay8/1(d)
  [unpack_recvd0] -> Inverter2/1
  Logical6/1 -> counter22/2
  Inverter5/1 -> Logical6/1
  [up_timestep_error_future] -> counter23/2
  [up_timestep_error_past] -> counter13/2
  Delay79/1(q) -> counter13/1, counter23/1, counter21/1, counter22/1, counter20/1
  counter23/1 -> Delay15/1(d)
  counter13/1 -> Delay30/1(d)
  pipeline67/1(q) -> [snappfb_dsel]
  control/18(in_snappfb_dsel) -> pipeline67/1(d)
  pipeline72/1(q) -> [snapcoarse_arm]
  control/16(in_snapcoarse_arm) -> pipeline72/1(d)
  pipeline77/1(q) -> [snapquant_arm]
  control/19(in_snapquant_arm) -> pipeline77/1(d)
  [up_gbe0] -> pipeline108/1(d)
  [up_gbe1] -> pipeline109/1(d)
  [up_gbe2] -> pipeline110/1(d)
  [up_gbe3] -> pipeline111/1(d)
  up_debug/1(in_gbe_timestep) -> Delay88/1(d)
  Delay88/1(q) -> [gbe_timestep]
  unpack_and_reorder/12(mcnt_relock) -> [unpack_mcnt_relock]
  [unpack_recvd0] -> Inverter6/1
  [unpack_en] -> Logical10/2
  Inverter6/1 -> Logical10/1
  Logical10/1 -> [unpack_missing0]
  [unpack_recvd1] -> Inverter7/1
  [unpack_en] -> Logical13/2
  Inverter7/1 -> Logical13/1
  Logical13/1 -> [unpack_missing1]
  pipeline61/1(q) -> [tvg_unpack_flags_en]
  control/22(in_tvg_unpack_flags_en) -> pipeline61/1(d)
  bus_expand17/1(msb_out2) -> [unpack_recvd0]
  bus_expand17/2(lsb_out1) -> [unpack_recvd1]
  [unpack_recvd1] -> Inverter5/1
  Slice12/1 -> [time80]
  impulse_gen0/3(dvalid) -> [valid80]
  impulse_gen0/1(sync_out) -> [sync80]
  impulse_gen0/2(dout) -> [d80_adc0]
  impulse_gen0/4(misco) -> Slice12/1
  [tvg_adc_en] -> impulse_gen0/1(tvg_en)
  impulse_gen1/1(sync_out) -> Terminator1/1
  impulse_gen1/2(dout) -> [d80_adc1]
  impulse_gen1/3(dvalid) -> Terminator2/1
  impulse_gen1/4(misco) -> [dig_flags]
  [tvg_adc_en] -> impulse_gen1/1(tvg_en)
  impulse0/1(in_offset) -> pipeline68/1(d)
  impulse0/2(in_amplitude) -> pipeline69/1(d)
  impulse1/1(in_offset) -> pipeline70/1(d)
  impulse1/2(in_amplitude) -> pipeline71/1(d)
  sync_gen/1(sync) -> impulse_gen0/4(sync_in), impulse_gen1/4(sync_in)
  bus_expand6/1(msb_out2) -> impulse_gen0/5(din)
  bus_expand6/2(lsb_out1) -> impulse_gen1/5(din)
  sync_gen/5(misco) -> impulse_gen1/7(misci)
  sync_gen/4(time_out) -> impulse_gen0/7(misci)
  pipeline63/1(q) -> unpack_and_reorder/4(en)
  pipeline62/1(q) -> unpack_and_reorder/3(eof)
  pipeline64/1(q) -> unpack_and_reorder/1(rst)
  pipeline68/1(q) -> impulse_gen0/2(impulse_offset)
  pipeline69/1(q) -> impulse_gen0/3(impulse_amplitude)
  pipeline70/1(q) -> impulse_gen1/2(impulse_offset)
  pipeline71/1(q) -> impulse_gen1/3(impulse_amplitude)
  Delay7/1(q) -> recverr_ctr/1(out_p0)
  Delay8/1(q) -> recverr_ctr/2(out_p1)
  Delay13/1(q) -> mcnt_relock/1(out_reg)
  Delay15/1(q) -> timestep_ages/1(out_future)
  Delay30/1(q) -> timestep_ages/2(out_past)
  pipeline93/1(q) -> gbe0/9(debug_rst)
  pipeline98/1(q) -> gbe2/9(debug_rst)
  pipeline99/1(q) -> gbe3/9(debug_rst)
  pipeline100/1(q) -> gbe1/9(debug_rst)
  pipeline101/1(q) -> gbe0/1(rst)
  pipeline102/1(q) -> gbe1/1(rst)
  pipeline103/1(q) -> gbe3/1(rst)
  pipeline104/1(q) -> gbe2/1(rst)
  iptx_base/1(in_reg) -> pipeline105/1(d)
  pipeline105/1(q) -> [tx_ip_base]
  tx_metadata/1(in_porttx) -> pipeline106/1(d)
  tx_metadata/2(in_board_id) -> pipeline107/1(d)
  pipeline106/1(q) -> [tx_port]
  pipeline107/1(q) -> [tx_board_id]
  pipeline108/1(q) -> gbe_status/1(out_gbe0_linkup)
  pipeline109/1(q) -> gbe_status/2(out_gbe1_linkup)
  pipeline110/1(q) -> gbe_status/3(out_gbe2_linkup)
  pipeline111/1(q) -> gbe_status/4(out_gbe3_linkup)
  pipeline112/1(q) -> sync_timestamp_msw/1(out_reg)
  pipeline113/1(q) -> sync_timestamp_lsw/1(out_time_lsw)
  pipeline114/1(q) -> sync_timestamp_lsw/2(out_pkt_size)
  pipeline115/1(q) -> sync_timestamp_lsw/3(out_tstep_err_ctr)
  pipeline116/1(q) -> sync_timestamp_lsw/4(out_sync80_ctr)
  pipeline117/1(q) -> sync_timestamp_lsw/5(out_valid80_ctr)
  Delay10/1 -> gbe0/2(tx_data)
  Delay11/1 -> gbe0/4(tx_dest_ip)
  Delay12/1 -> gbe0/5(tx_dest_port)
  Delay14/1 -> gbe2/2(tx_data)
  Delay21/1 -> gbe2/5(tx_dest_port)
  Delay20/1 -> gbe2/4(tx_dest_ip)
  Delay24/1 -> gbe3/5(tx_dest_port)
  Delay23/1 -> gbe3/4(tx_dest_ip)
  Delay22/1 -> gbe3/2(tx_data)
  Delay27/1 -> gbe1/5(tx_dest_port)
  Delay26/1 -> gbe1/4(tx_dest_ip)
  Delay25/1 -> gbe1/2(tx_data)
  Logical/1 -> gbe0/3(tx_valid)
  Logical2/1 -> gbe1/3(tx_valid)
  Logical3/1 -> gbe3/3(tx_valid)
  Logical8/1 -> gbe2/3(tx_valid)
  [gbe_txen] -> gbe1/6(tx_end_of_frame), Logical2/1
  Constant6/1 -> Logical/2
  [gbe_txen] -> gbe3/6(tx_end_of_frame), Logical3/1
  [gbe_txen] -> gbe2/6(tx_end_of_frame), Logical8/1
  [gbe_txen] -> gbe0/6(tx_end_of_frame), Logical/1
  [clr_status] -> tl_unpack_flags/1(rst)
  [unpack_en] -> tl_unpack_flags/4(en)
  Constant1/1 -> tl_unpack_flags/3(load_value)
  tl_unpack_flags/5(misco) -> bus_expand11/1(bus_in)
  tl_unpack_flags/1(value) -> Terminator13/1
  Concat10/1 -> pipeline81/1(d)
  [tvg_unpack_flags_en] -> flag_mux0/1(tvg_en)
  tl_unpack_flags/2(enable) -> flag_mux0/2(ld_val)
  tl_unpack_flags/3(dvalid) -> flag_mux0/3(en)
  bus_expand11/2(lsb_out1) -> flag_mux0/5(flag)
  pipeline81/1(q) -> flag_mux0/6(tvg_flag)
  Constant31/1 -> Concat9/2
  Concat9/1 -> tl_unpack_flags/2(current_time)
  Concat11/1 -> tl_unpack_flags/5(misci)
  [unpack_timestamp] -> Concat9/1
  [tvg_d80_en] -> en_gen/5(tvg_en)
  pipeline122/1(q) -> [tvg_pfb_flags_en]
  control/23(in_tvg_pfb_flags_en) -> pipeline122/1(d)
  tl_unpack_flags/4(time) -> Concat/1
  bus_expand11/1(msb_out2) -> Concat/2
  Concat/1 -> flag_mux0/4(misci)
  flag_mux0/1(dvalid) -> en_gen/1(en)
  flag_mux0/2(misco) -> bus_expand1/1(bus_in)
  bus_expand1/1(msb_out2) -> en_gen/2(time_in)
  bus_expand1/2(lsb_out1) -> en_gen/3(din)
  flag_mux0/3(flags_out) -> en_gen/4(misci)
  unpack_and_reorder/6(flags) -> bus_expand2/1(bus_in)
  bus_expand2/1(msb_out4) -> [unpack_ndiode0]
  bus_expand2/2(out3) -> [unpack_adc_or0]
  bus_expand2/3(out2) -> [unpack_ndiode1]
  [unpack_fifo_pktof] -> Concat11/7
  [unpack_spead_error] -> Concat11/9
  [unpack_discarding] -> Concat11/6
  [unpack_mcnt_relock] -> Concat11/5
  [unpack_adc_or1] -> Concat11/11
  [unpack_missing1] -> Concat11/4
  [unpack_fifo_of] -> Concat11/8
  [unpack_ndiode0] -> Concat11/12
  [unpack_ndiode1] -> Concat11/13
  [unpack_adc_or0] -> Concat11/10
  [unpack_missing0] -> Concat11/3
  [timestep_error] -> Concat11/2
  [unpack_d80] -> Concat11/1
  unpack_and_reorder/7(fifo_of) -> Relational3/1
  Constant8/1 -> Relational3/2
  Relational3/1 -> [unpack_fifo_of]
  Constant34/1 -> Relational4/2
  unpack_and_reorder/8(packet_of) -> Relational4/1
  Relational4/1 -> [unpack_fifo_pktof]
  Constant35/1 -> Relational5/2
  unpack_and_reorder/9(spead_error) -> Relational5/1
  Relational5/1 -> [unpack_spead_error]
  unpack_flags/9(in_adc_or0) -> Concat10/9
  unpack_flags/2(in_missing0) -> Concat10/2
  unpack_flags/8(in_spead_error) -> Concat10/8
  unpack_flags/6(in_pktof) -> Concat10/6
  unpack_flags/10(in_adc_or1) -> Concat10/10
  unpack_flags/7(in_fifo_of) -> Concat10/7
  unpack_flags/4(in_mcnt_relock) -> Concat10/4
  unpack_flags/11(in_ndiode0) -> Concat10/11
  unpack_flags/1(in_timestep_error) -> Concat10/1
  unpack_flags/5(in_discarded) -> Concat10/5
  unpack_flags/12(in_ndiode1) -> Concat10/12
  unpack_flags/3(in_missing1) -> Concat10/3
  Constant13/1 -> Delay26/1
  Constant14/1 -> Delay27/1
  Constant12/1 -> Logical2/2
  Constant11/1 -> Delay25/1
  Constant15/1 -> Delay14/1
  Constant17/1 -> Logical8/2
  Constant18/1 -> Delay20/1
  Constant21/1 -> Delay21/1
  Constant26/1 -> Delay23/1
  Constant27/1 -> Delay24/1
  Constant24/1 -> Logical3/2
  Constant22/1 -> Delay22/1
  Constant28/1 -> snapshot/2(we)
  Constant29/1 -> snapshot/3(trig)
  [d80_adc0] -> Reinterpret/1
  Slice2/1 -> Concat1/1
  Slice3/1 -> Concat1/2
  Concat1/1 -> Mux/3
  Slice1/1 -> Mux/2
  Slice4/1 -> Concat3/1
  Slice5/1 -> Concat3/2
  Concat3/1 -> Mux/4
  Slice6/1 -> Concat4/1
  Slice8/1 -> Concat4/2
  Concat4/1 -> Mux/5
  Reinterpret/1 -> Slice2/1, Delay4/1, Slice4/1, Slice6/1, Delay2/1, Delay3/1, Delay1/1, Slice1/1
  Slice13/1 -> Mux/6
  Delay3/1 -> Slice13/1
  Delay4/1 -> Slice3/1
  Mux/1 -> snapshot/1(din)
  Delay1/1 -> Slice5/1
  Delay2/1 -> Slice8/1
  [valid80] -> Assert/1
  Assert/1 -> Counter/1
  Constant2/1 -> snapshot1/2(we)
  Constant16/1 -> snapshot1/3(trig)
  [d80_adc1] -> Reinterpret1/1
  Slice18/1 -> Concat5/1
  Slice19/1 -> Concat5/2
  Concat5/1 -> Mux1/3
  Slice15/1 -> Mux1/2
  Slice21/1 -> Concat7/1
  Slice22/1 -> Concat7/2
  Concat7/1 -> Mux1/4
  Slice23/1 -> Concat8/1
  Slice24/1 -> Concat8/2
  Concat8/1 -> Mux1/5
  Slice17/1 -> Mux1/6
  Delay9/1 -> Slice17/1
  Delay16/1 -> Slice19/1
  Mux1/1 -> snapshot1/1(din)
  Delay5/1 -> Slice22/1
  Delay6/1 -> Slice24/1
  Reinterpret1/1 -> Delay5/1, Slice23/1, Delay9/1, Delay6/1, Slice21/1, Delay16/1, Slice18/1, Slice15/1
  Counter/1 -> Mux/1, Mux1/1
